simulink library "halin"  (R2021b)
settings: Solver=VariableStepAuto  StartTime=0.0  StopTime=10.0  RelTol=1e-3
undefined symbols (not defined in the file): TRUE
libraries: FVT_lib x177, hcu_lib x55
(part 17 of 17)

== system halin/HAL_IN/CAN4/zGW_SEAT1/PSEATSWVer ==
  PSEAT_SW_Ver : Inport
  UnitConverter : DataTypeConversion  OutDataTypeStr=uint16
  VHAL_PSEATSWVer_enum : Outport
  wires:
  UnitConverter/1 -> VHAL_PSEATSWVer_enum/1
  PSEAT_SW_Ver/1 -> UnitConverter/1

== system halin/HAL_IN/CAN4/zGW_SEAT1/PSEATVentSta ==
  PSEAT_Vent_Sta : Inport
  UnitConverter : DataTypeConversion  OutDataTypeStr=uint8
  VHAL_PSEATVentSta_enum : Outport
  wires:
  UnitConverter/1 -> VHAL_PSEATVentSta_enum/1
  PSEAT_Vent_Sta/1 -> UnitConverter/1

== system halin/HAL_IN/CAN4/zGW_SEAT1/PSEATheatersta ==
  PSEAT_heater_sta : Inport
  UnitConverter : DataTypeConversion  OutDataTypeStr=uint8
  VHAL_PSEATheatersta_enum : Outport
  wires:
  UnitConverter/1 -> VHAL_PSEATheatersta_enum/1
  PSEAT_heater_sta/1 -> UnitConverter/1

== system halin/HAL_IN/CAN5/TBOX1/CbnPreACEnaReq ==
  CbnPreACEnaReq : Inport
  UnitConverter : DataTypeConversion  OutDataTypeStr=uint8
  VHAL_CbnPreACEnaReq_enum : Outport
  wires:
  UnitConverter/1 -> VHAL_CbnPreACEnaReq_enum/1
  CbnPreACEnaReq/1 -> UnitConverter/1

== system halin/HAL_IN/CAN5/TBOX1/PowerOffTSet ==
  PowerOff_T_Set : Inport
  UnitConverter : DataTypeConversion  OutDataTypeStr=uint8
  convert_in : FVT_lib/hal/convert_in  gain=1  offset=1
  VHAL_PowerOffTSet_cnt : Outport
  wires:
  convert_in/1 -> VHAL_PowerOffTSet_cnt/1
  UnitConverter/1 -> convert_in/1
  PowerOff_T_Set/1 -> UnitConverter/1

== system halin/HAL_IN/CAN5/TBOX1/ReDoorLock ==
  Re_DoorLock : Inport
  UnitConverter : DataTypeConversion  OutDataTypeStr=uint16
  VHAL_ReDoorLock_enum : Outport
  wires:
  UnitConverter/1 -> VHAL_ReDoorLock_enum/1
  Re_DoorLock/1 -> UnitConverter/1

== system halin/HAL_IN/CAN5/TBOX1/ReOutsideMirror ==
  ReOutsideMirror : Inport
  UnitConverter : DataTypeConversion  OutDataTypeStr=uint8
  VHAL_ReOutsideMirror_enum : Outport
  wires:
  UnitConverter/1 -> VHAL_ReOutsideMirror_enum/1
  ReOutsideMirror/1 -> UnitConverter/1

== system halin/HAL_IN/CAN5/TBOX1/RePwrReqTbox ==
  Re_PwrReqTbox : Inport
  UnitConverter : DataTypeConversion  OutDataTypeStr=uint8
  VHAL_RePwrReqTbox_enum : Outport
  wires:
  UnitConverter/1 -> VHAL_RePwrReqTbox_enum/1
  Re_PwrReqTbox/1 -> UnitConverter/1

== system halin/HAL_IN/CAN5/TBOX1/ReRadio ==
  Re_Radio : Inport
  UnitConverter : DataTypeConversion  OutDataTypeStr=uint8
  VHAL_ReRadio_flg : Outport
  wires:
  UnitConverter/1 -> VHAL_ReRadio_flg/1
  Re_Radio/1 -> UnitConverter/1

== system halin/HAL_IN/CAN5/TBOX1/RemoteACTemp ==
  Remote_ACTemp : Inport
  UnitConverter : DataTypeConversion  OutDataTypeStr=uint8
  convert_in : FVT_lib/hal/convert_in  gain=0.5  offset=17
  VHAL_RemoteACTemp_C : Outport
  wires:
  convert_in/1 -> VHAL_RemoteACTemp_C/1
  UnitConverter/1 -> convert_in/1
  Remote_ACTemp/1 -> UnitConverter/1

== system halin/HAL_IN/CAN5/TBOX1/RemoteAutoReq ==
  Remote_AutoReq : Inport
  UnitConverter : DataTypeConversion  OutDataTypeStr=uint8
  VHAL_RemoteAutoReq_flg : Outport
  wires:
  UnitConverter/1 -> VHAL_RemoteAutoReq_flg/1
  Remote_AutoReq/1 -> UnitConverter/1

== system halin/HAL_IN/CAN5/TBOX1/TBOXNETSIGSTR ==
  TBOX_NET_SIG_STR : Inport
  UnitConverter : DataTypeConversion  OutDataTypeStr=uint8
  VHAL_TBOXNETSIGSTR_enum : Outport
  wires:
  UnitConverter/1 -> VHAL_TBOXNETSIGSTR_enum/1
  TBOX_NET_SIG_STR/1 -> UnitConverter/1

== system halin/HAL_IN/CAN5/TBOX1/TBOXRemotePW ==
  TBOX_Remote_PW : Inport
  UnitConverter : DataTypeConversion  OutDataTypeStr=uint8
  VHAL_TBOXRemotePW_enum : Outport
  wires:
  UnitConverter/1 -> VHAL_TBOXRemotePW_enum/1
  TBOX_Remote_PW/1 -> UnitConverter/1

== system halin/HAL_IN/CAN5/TBOX1/TBOXTESTSTATUS ==
  TBOX_TEST_STATUS : Inport
  UnitConverter : DataTypeConversion  OutDataTypeStr=uint8
  VHAL_TBOXTESTSTATUS_enum : Outport
  wires:
  UnitConverter/1 -> VHAL_TBOXTESTSTATUS_enum/1
  TBOX_TEST_STATUS/1 -> UnitConverter/1

== system halin/HAL_IN/CAN5/TBOX2/TimeSyncFromBSDay ==
  TimeSyncFromBS_Day : Inport
  UnitConverter : DataTypeConversion  OutDataTypeStr=uint8
  VHAL_TimeSyncFromBSDay_DAY : Outport
  wires:
  UnitConverter/1 -> VHAL_TimeSyncFromBSDay_DAY/1
  TimeSyncFromBS_Day/1 -> UnitConverter/1

== system halin/HAL_IN/CAN5/TBOX2/TimeSyncFromBSHour ==
  TimeSyncFromBS_Hour : Inport
  UnitConverter : DataTypeConversion  OutDataTypeStr=uint8
  VHAL_TimeSyncFromBSHour_hr : Outport
  wires:
  UnitConverter/1 -> VHAL_TimeSyncFromBSHour_hr/1
  TimeSyncFromBS_Hour/1 -> UnitConverter/1

== system halin/HAL_IN/CAN5/TBOX2/TimeSyncFromBSMinute ==
  TimeSyncFromBS_Minute : Inport
  UnitConverter : DataTypeConversion  OutDataTypeStr=uint8
  VHAL_TimeSyncFromBSMinute_min : Outport
  wires:
  UnitConverter/1 -> VHAL_TimeSyncFromBSMinute_min/1
  TimeSyncFromBS_Minute/1 -> UnitConverter/1

== system halin/HAL_IN/CAN5/TBOX2/TimeSyncFromBSMonth ==
  TimeSyncFromBS_Month : Inport
  UnitConverter : DataTypeConversion  OutDataTypeStr=uint8
  VHAL_TimeSyncFromBSMonth_MONTH : Outport
  wires:
  UnitConverter/1 -> VHAL_TimeSyncFromBSMonth_MONTH/1
  TimeSyncFromBS_Month/1 -> UnitConverter/1

== system halin/HAL_IN/CAN5/TBOX2/TimeSyncFromBSSecond ==
  TimeSyncFromBS_Second : Inport
  UnitConverter : DataTypeConversion  OutDataTypeStr=uint8
  VHAL_TimeSyncFromBSSecond_s : Outport
  wires:
  UnitConverter/1 -> VHAL_TimeSyncFromBSSecond_s/1
  TimeSyncFromBS_Second/1 -> UnitConverter/1

== system halin/HAL_IN/CAN5/TBOX2/TimeSyncFromBSYear ==
  TimeSyncFromBS_Year : Inport
  UnitConverter : DataTypeConversion  OutDataTypeStr=uint8
  convert_in : FVT_lib/hal/convert_in  gain=1  offset=2000
  VHAL_TimeSyncFromBSYear_YEAR : Outport
  wires:
  convert_in/1 -> VHAL_TimeSyncFromBSYear_YEAR/1
  UnitConverter/1 -> convert_in/1
  TimeSyncFromBS_Year/1 -> UnitConverter/1

== system halin/HAL_IN/CAN5/TBOX3/ChargePercentSet ==
  Charge_Percent_Set : Inport
  UnitConverter : DataTypeConversion  OutDataTypeStr=uint8
  VHAL_ChargePercentSet_pct : Outport
  wires:
  UnitConverter/1 -> VHAL_ChargePercentSet_pct/1
  Charge_Percent_Set/1 -> UnitConverter/1

== system halin/HAL_IN/CAN5/TBOX3/ReserveChargeOFFDay ==
  ReserveChargeOFF_Day : Inport
  UnitConverter : DataTypeConversion  OutDataTypeStr=uint8
  VHAL_ReserveChargeOFFDay_DAY : Outport
  wires:
  UnitConverter/1 -> VHAL_ReserveChargeOFFDay_DAY/1
  ReserveChargeOFF_Day/1 -> UnitConverter/1

== system halin/HAL_IN/CAN5/TBOX3/ReserveChargeOFFHour ==
  ReserveChargeOFF_Hour : Inport
  UnitConverter : DataTypeConversion  OutDataTypeStr=uint8
  VHAL_ReserveChargeOFFHour_hr : Outport
  wires:
  UnitConverter/1 -> VHAL_ReserveChargeOFFHour_hr/1
  ReserveChargeOFF_Hour/1 -> UnitConverter/1

== system halin/HAL_IN/CAN5/TBOX3/ReserveChargeOFFMinute ==
  ReserveChargeOFF_Minute : Inport
  UnitConverter : DataTypeConversion  OutDataTypeStr=uint8
  VHAL_ReserveChargeOFFMinute_min : Outport
  wires:
  UnitConverter/1 -> VHAL_ReserveChargeOFFMinute_min/1
  ReserveChargeOFF_Minute/1 -> UnitConverter/1

== system halin/HAL_IN/CAN5/TBOX3/ReserveChargeOFFMonth ==
  ReserveChargeOFF_Month : Inport
  UnitConverter : DataTypeConversion  OutDataTypeStr=uint8
  VHAL_ReserveChargeOFFMonth_MONTH : Outport
  wires:
  UnitConverter/1 -> VHAL_ReserveChargeOFFMonth_MONTH/1
  ReserveChargeOFF_Month/1 -> UnitConverter/1

== system halin/HAL_IN/CAN5/TBOX3/ReserveChargeOFFYear ==
  ReserveChargeOFF_Year : Inport
  UnitConverter : DataTypeConversion  OutDataTypeStr=uint8
  convert_in : FVT_lib/hal/convert_in  gain=1  offset=2000
  VHAL_ReserveChargeOFFYear_YEAR : Outport
  wires:
  convert_in/1 -> VHAL_ReserveChargeOFFYear_YEAR/1
  UnitConverter/1 -> convert_in/1
  ReserveChargeOFF_Year/1 -> UnitConverter/1

== system halin/HAL_IN/CAN5/TBOX3/ReserveChargeOnDay ==
  ReserveChargeOn_Day : Inport
  UnitConverter : DataTypeConversion  OutDataTypeStr=uint8
  VHAL_ReserveChargeOnDay_DAY : Outport
  wires:
  UnitConverter/1 -> VHAL_ReserveChargeOnDay_DAY/1
  ReserveChargeOn_Day/1 -> UnitConverter/1

== system halin/HAL_IN/CAN5/TBOX3/ReserveChargeOnHour ==
  ReserveChargeOn_Hour : Inport
  UnitConverter : DataTypeConversion  OutDataTypeStr=uint8
  VHAL_ReserveChargeOnHour_hr : Outport
  wires:
  UnitConverter/1 -> VHAL_ReserveChargeOnHour_hr/1
  ReserveChargeOn_Hour/1 -> UnitConverter/1

== system halin/HAL_IN/CAN5/TBOX3/ReserveChargeOnMinute ==
  ReserveChargeOn_Minute : Inport
  UnitConverter : DataTypeConversion  OutDataTypeStr=uint8
  VHAL_ReserveChargeOnMinute_min : Outport
  wires:
  UnitConverter/1 -> VHAL_ReserveChargeOnMinute_min/1
  ReserveChargeOn_Minute/1 -> UnitConverter/1

== system halin/HAL_IN/CAN5/TBOX3/ReserveChargeOnMonth ==
  ReserveChargeOn_Month : Inport
  UnitConverter : DataTypeConversion  OutDataTypeStr=uint8
  VHAL_ReserveChargeOnMonth_MONTH : Outport
  wires:
  UnitConverter/1 -> VHAL_ReserveChargeOnMonth_MONTH/1
  ReserveChargeOn_Month/1 -> UnitConverter/1

== system halin/HAL_IN/CAN5/TBOX3/ReserveChargeOnYear ==
  ReserveChargeOn_Year : Inport
  UnitConverter : DataTypeConversion  OutDataTypeStr=uint8
  convert_in : FVT_lib/hal/convert_in  gain=1  offset=2000
  VHAL_ReserveChargeOnYear_YEAR : Outport
  wires:
  convert_in/1 -> VHAL_ReserveChargeOnYear_YEAR/1
  UnitConverter/1 -> convert_in/1
  ReserveChargeOn_Year/1 -> UnitConverter/1

== system halin/HAL_IN/CAN5/TBOX3/TBOXHWVER ==
  TBOX_HW_VER : Inport
  UnitConverter : DataTypeConversion  OutDataTypeStr=uint32
  VHAL_TBOXHWVER_enum : Outport
  wires:
  UnitConverter/1 -> VHAL_TBOXHWVER_enum/1
  TBOX_HW_VER/1 -> UnitConverter/1

== system halin/HAL_IN/CAN5/TBOX3/TBOXSWVER ==
  TBOX_SW_VER : Inport
  UnitConverter : DataTypeConversion  OutDataTypeStr=uint32
  VHAL_TBOXSWVER_enum : Outport
  wires:
  UnitConverter/1 -> VHAL_TBOXSWVER_enum/1
  TBOX_SW_VER/1 -> UnitConverter/1

== system halin/HAL_IN/CAN6/FCM1/ACCComfortBandLower ==
  ACC_ComfortBandLower : Inport
  UnitConverter : DataTypeConversion  OutDataTypeStr=uint16
  convert_in : FVT_lib/hal/convert_in  gain=0.05  offset=-15
  VHAL_ACCComfortBandLower_mps2 : Outport
  wires:
  convert_in/1 -> VHAL_ACCComfortBandLower_mps2/1
  UnitConverter/1 -> convert_in/1
  ACC_ComfortBandLower/1 -> UnitConverter/1

== system halin/HAL_IN/CAN6/FCM1/ACCComfortBandUpper ==
  ACC_ComfortBandUpper : Inport
  UnitConverter : DataTypeConversion  OutDataTypeStr=uint16
  convert_in : FVT_lib/hal/convert_in  gain=0.05  offset=-15
  VHAL_ACCComfortBandUpper_mps2 : Outport
  wires:
  convert_in/1 -> VHAL_ACCComfortBandUpper_mps2/1
  UnitConverter/1 -> convert_in/1
  ACC_ComfortBandUpper/1 -> UnitConverter/1

== system halin/HAL_IN/CAN6/FCM1/ACCJerkLowerLimit ==
  ACC_JerkLowerLimit : Inport
  UnitConverter : DataTypeConversion  OutDataTypeStr=uint8
  convert_in : FVT_lib/hal/convert_in  gain=0.1  offset=-6
  VHAL_ACCJerkLowerLimit_mps3 : Outport
  wires:
  convert_in/1 -> VHAL_ACCJerkLowerLimit_mps3/1
  UnitConverter/1 -> convert_in/1
  ACC_JerkLowerLimit/1 -> UnitConverter/1

== system halin/HAL_IN/CAN6/FCM1/ACCJerkUpperLimit ==
  ACC_JerkUpperLimit : Inport
  UnitConverter : DataTypeConversion  OutDataTypeStr=uint8
  convert_in : FVT_lib/hal/convert_in  gain=0.1  offset=-6
  VHAL_ACCJerkUpperLimit_mps3 : Outport
  wires:
  convert_in/1 -> VHAL_ACCJerkUpperLimit_mps3/1
  UnitConverter/1 -> convert_in/1
  ACC_JerkUpperLimit/1 -> UnitConverter/1

== system halin/HAL_IN/CAN6/FCM1/ACCObjDist ==
  ACC_ObjDist : Inport
  UnitConverter : DataTypeConversion  OutDataTypeStr=uint16
  convert_in : FVT_lib/hal/convert_in  gain=0.1  offset=0
  VHAL_ACCObjDist_m : Outport
  wires:
  convert_in/1 -> VHAL_ACCObjDist_m/1
  UnitConverter/1 -> convert_in/1
  ACC_ObjDist/1 -> UnitConverter/1

== system halin/HAL_IN/CAN6/FCM1/ACCObjDstLvl ==
  ACC_ObjDstLvl : Inport
  UnitConverter : DataTypeConversion  OutDataTypeStr=uint8
  VHAL_ACCObjDstLvl_enum : Outport
  wires:
  UnitConverter/1 -> VHAL_ACCObjDstLvl_enum/1
  ACC_ObjDstLvl/1 -> UnitConverter/1

== system halin/HAL_IN/CAN6/FCM1/ACCObjRelSpd ==
  ACC_ObjRelSpd : Inport
  UnitConverter : DataTypeConversion  OutDataTypeStr=uint16
  convert_in : FVT_lib/hal/convert_in  gain=0.1  offset=-100
  VHAL_ACCObjRelSpd_mps : Outport
  wires:
  convert_in/1 -> VHAL_ACCObjRelSpd_mps/1
  UnitConverter/1 -> convert_in/1
  ACC_ObjRelSpd/1 -> UnitConverter/1

== system halin/HAL_IN/CAN6/FCM1/ACCRequiredAccel ==
  ACC_RequiredAccel : Inport
  UnitConverter : DataTypeConversion  OutDataTypeStr=uint16
  convert_in : FVT_lib/hal/convert_in  gain=0.05  offset=-15
  VHAL_ACCRequiredAccel_mps2 : Outport
  wires:
  convert_in/1 -> VHAL_ACCRequiredAccel_mps2/1
  UnitConverter/1 -> convert_in/1
  ACC_RequiredAccel/1 -> UnitConverter/1

== system halin/HAL_IN/CAN6/FCM1/ACCTakeoverReq ==
  ACC_TakeoverReq : Inport
  UnitConverter : DataTypeConversion  OutDataTypeStr=uint8
  VHAL_ACCTakeoverReq_flg : Outport
  wires:
  UnitConverter/1 -> VHAL_ACCTakeoverReq_flg/1
  ACC_TakeoverReq/1 -> UnitConverter/1

== system halin/HAL_IN/CAN6/FCM1/ACCVehHoldReq ==
  ACC_VehHoldReq : Inport
  UnitConverter : DataTypeConversion  OutDataTypeStr=uint8
  VHAL_ACCVehHoldReq_flg : Outport
  wires:
  UnitConverter/1 -> VHAL_ACCVehHoldReq_flg/1
  ACC_VehHoldReq/1 -> UnitConverter/1

== system halin/HAL_IN/CAN6/FCM1/ADASACCSta ==
  ADAS_ACC_Sta : Inport
  UnitConverter : DataTypeConversion  OutDataTypeStr=uint8
  VHAL_ADASACCSta_enum : Outport
  wires:
  UnitConverter/1 -> VHAL_ADASACCSta_enum/1
  ADAS_ACC_Sta/1 -> UnitConverter/1

== system halin/HAL_IN/CAN6/FCM1/ADASAEBReq ==
  ADAS_AEBReq : Inport
  UnitConverter : DataTypeConversion  OutDataTypeStr=uint8
  VHAL_ADASAEBReq_enum : Outport
  wires:
  UnitConverter/1 -> VHAL_ADASAEBReq_enum/1
  ADAS_AEBReq/1 -> UnitConverter/1

== system halin/HAL_IN/CAN6/FCM1/ADASAEBSta ==
  ADAS_AEB_Sta : Inport
  UnitConverter : DataTypeConversion  OutDataTypeStr=uint8
  VHAL_ADASAEBSta_enum : Outport
  wires:
  UnitConverter/1 -> VHAL_ADASAEBSta_enum/1
  ADAS_AEB_Sta/1 -> UnitConverter/1

== system halin/HAL_IN/CAN6/FCM1/ADASCAMSpdLim ==
  ADAS_CAM_SpdLim : Inport
  UnitConverter : DataTypeConversion  OutDataTypeStr=uint8
  VHAL_ADASCAMSpdLim_enum : Outport
  wires:
  UnitConverter/1 -> VHAL_ADASCAMSpdLim_enum/1
  ADAS_CAM_SpdLim/1 -> UnitConverter/1

== system halin/HAL_IN/CAN6/FCM1/ADASDBSReq ==
  ADAS_DBSReq : Inport
  UnitConverter : DataTypeConversion  OutDataTypeStr=uint8
  VHAL_ADASDBSReq_enum : Outport
  wires:
  UnitConverter/1 -> VHAL_ADASDBSReq_enum/1
  ADAS_DBSReq/1 -> UnitConverter/1

== system halin/HAL_IN/CAN6/FCM1/ADASFCWMute ==
  ADAS_FCW_Mute : Inport
  UnitConverter : DataTypeConversion  OutDataTypeStr=uint8
  VHAL_ADASFCWMute_flg : Outport
  wires:
  UnitConverter/1 -> VHAL_ADASFCWMute_flg/1
  ADAS_FCW_Mute/1 -> UnitConverter/1

== system halin/HAL_IN/CAN6/FCM1/ADASFCWSta ==
  ADAS_FCW_Sta : Inport
  UnitConverter : DataTypeConversion  OutDataTypeStr=uint8
  VHAL_ADASFCWSta_enum : Outport
  wires:
  UnitConverter/1 -> VHAL_ADASFCWSta_enum/1
  ADAS_FCW_Sta/1 -> UnitConverter/1

== system halin/HAL_IN/CAN6/FCM1/ADASFaultSta ==
  ADAS_FaultSta : Inport
  UnitConverter : DataTypeConversion  OutDataTypeStr=uint8
  VHAL_ADASFaultSta_flg : Outport
  wires:
  UnitConverter/1 -> VHAL_ADASFaultSta_flg/1
  ADAS_FaultSta/1 -> UnitConverter/1

== system halin/HAL_IN/CAN6/FCM1/ADASFltWrnReq ==
  ADAS_FltWrnReq : Inport
  UnitConverter : DataTypeConversion  OutDataTypeStr=uint8
  VHAL_ADASFltWrnReq_flg : Outport
  wires:
  UnitConverter/1 -> VHAL_ADASFltWrnReq_flg/1
  ADAS_FltWrnReq/1 -> UnitConverter/1

== system halin/HAL_IN/CAN6/FCM1/ADASForceIdle ==
  ADAS_ForceIdle : Inport
  UnitConverter : DataTypeConversion  OutDataTypeStr=uint8
  VHAL_ADASForceIdle_flg : Outport
  wires:
  UnitConverter/1 -> VHAL_ADASForceIdle_flg/1
  ADAS_ForceIdle/1 -> UnitConverter/1

== system halin/HAL_IN/CAN6/FCM1/ADASISASta ==
  ADAS_ISA_Sta : Inport
  UnitConverter : DataTypeConversion  OutDataTypeStr=uint8
  VHAL_ADASISASta_enum : Outport
  wires:
  UnitConverter/1 -> VHAL_ADASISASta_enum/1
  ADAS_ISA_Sta/1 -> UnitConverter/1

== system halin/HAL_IN/CAN6/FCM1/ADASLDWMute ==
  ADAS_LDW_Mute : Inport
  UnitConverter : DataTypeConversion  OutDataTypeStr=uint8
  VHAL_ADASLDWMute_flg : Outport
  wires:
  UnitConverter/1 -> VHAL_ADASLDWMute_flg/1
  ADAS_LDW_Mute/1 -> UnitConverter/1

== system halin/HAL_IN/CAN6/FCM1/ADASLDWSta ==
  ADAS_LDW_Sta : Inport
  UnitConverter : DataTypeConversion  OutDataTypeStr=uint8
  VHAL_ADASLDWSta_enum : Outport
  wires:
  UnitConverter/1 -> VHAL_ADASLDWSta_enum/1
  ADAS_LDW_Sta/1 -> UnitConverter/1

== system halin/HAL_IN/CAN6/FCM1/ADASLFCHandsOffWarning ==
  ADAS_LFC_Hands_Off_Warning : Inport
  UnitConverter : DataTypeConversion  OutDataTypeStr=uint8
  VHAL_ADASLFCHandsOffWarning_enum : Outport
  wires:
  UnitConverter/1 -> VHAL_ADASLFCHandsOffWarning_enum/1
  ADAS_LFC_Hands_Off_Warning/1 -> UnitConverter/1

== system halin/HAL_IN/CAN6/FCM1/ADASLFCSta ==
  ADAS_LFC_Sta : Inport
  UnitConverter : DataTypeConversion  OutDataTypeStr=uint8
  VHAL_ADASLFCSta_enum : Outport
  wires:
  UnitConverter/1 -> VHAL_ADASLFCSta_enum/1
  ADAS_LFC_Sta/1 -> UnitConverter/1

== system halin/HAL_IN/CAN6/FCM1/ADASLFCWarnSound ==
  ADAS_LFC_Warn_Sound : Inport
  UnitConverter : DataTypeConversion  OutDataTypeStr=uint16
  VHAL_ADASLFCWarnSound_enum : Outport
  wires:
  UnitConverter/1 -> VHAL_ADASLFCWarnSound_enum/1
  ADAS_LFC_Warn_Sound/1 -> UnitConverter/1

== system halin/HAL_IN/CAN6/FCM1/ADASLKASta ==
  ADAS_LKA_Sta : Inport
  UnitConverter : DataTypeConversion  OutDataTypeStr=uint16
  VHAL_ADASLKASta_enum : Outport
  wires:
  UnitConverter/1 -> VHAL_ADASLKASta_enum/1
  ADAS_LKA_Sta/1 -> UnitConverter/1

== system halin/HAL_IN/CAN6/FCM1/ADASLaneModeL ==
  ADAS_LaneModeL : Inport
  UnitConverter : DataTypeConversion  OutDataTypeStr=uint16
  VHAL_ADASLaneModeL_enum : Outport
  wires:
  UnitConverter/1 -> VHAL_ADASLaneModeL_enum/1
  ADAS_LaneModeL/1 -> UnitConverter/1

== system halin/HAL_IN/CAN6/FCM1/ADASLaneModeR ==
  ADAS_LaneModeR : Inport
  UnitConverter : DataTypeConversion  OutDataTypeStr=uint8
  VHAL_ADASLaneModeR_enum : Outport
  wires:
  UnitConverter/1 -> VHAL_ADASLaneModeR_enum/1
  ADAS_LaneModeR/1 -> UnitConverter/1

== system halin/HAL_IN/CAN6/FCM1/ADASLanecurveL ==
  ADAS_Lane_curveL : Inport
  UnitConverter : DataTypeConversion  OutDataTypeStr=uint8
  convert_in : FVT_lib/hal/convert_in  gain=0.0005  offset=-0.03
  VHAL_ADASLanecurveL_raw32 : Outport
  wires:
  convert_in/1 -> VHAL_ADASLanecurveL_raw32/1
  UnitConverter/1 -> convert_in/1
  ADAS_Lane_curveL/1 -> UnitConverter/1

== system halin/HAL_IN/CAN6/FCM1/ADASLanecurveR ==
  ADAS_Lane_curveR : Inport
  UnitConverter : DataTypeConversion  OutDataTypeStr=uint8
  convert_in : FVT_lib/hal/convert_in  gain=0.0005  offset=-0.03
  VHAL_ADASLanecurveR_raw32 : Outport
  wires:
  convert_in/1 -> VHAL_ADASLanecurveR_raw32/1
  UnitConverter/1 -> convert_in/1
  ADAS_Lane_curveR/1 -> UnitConverter/1

== system halin/HAL_IN/CAN6/FCM1/ADASLanetypeL ==
  ADAS_LanetypeL : Inport
  UnitConverter : DataTypeConversion  OutDataTypeStr=uint16
  VHAL_ADASLanetypeL_enum : Outport
  wires:
  UnitConverter/1 -> VHAL_ADASLanetypeL_enum/1
  ADAS_LanetypeL/1 -> UnitConverter/1

== system halin/HAL_IN/CAN6/FCM1/ADASLanetypeR ==
  ADAS_LanetypeR : Inport
  UnitConverter : DataTypeConversion  OutDataTypeStr=uint8
  VHAL_ADASLanetypeR_enum : Outport
  wires:
  UnitConverter/1 -> VHAL_ADASLanetypeR_enum/1
  ADAS_LanetypeR/1 -> UnitConverter/1

== system halin/HAL_IN/CAN6/FCM1/ADASSLIFSpdLim ==
  ADAS_SLIF_SpdLim : Inport
  UnitConverter : DataTypeConversion  OutDataTypeStr=uint8
  VHAL_ADASSLIFSpdLim_enum : Outport
  wires:
  UnitConverter/1 -> VHAL_ADASSLIFSpdLim_enum/1
  ADAS_SLIF_SpdLim/1 -> UnitConverter/1

== system halin/HAL_IN/CAN6/FCM1/ADASSLIFSta ==
  ADAS_SLIF_Sta : Inport
  UnitConverter : DataTypeConversion  OutDataTypeStr=uint8
  VHAL_ADASSLIFSta_enum : Outport
  wires:
  UnitConverter/1 -> VHAL_ADASSLIFSta_enum/1
  ADAS_SLIF_Sta/1 -> UnitConverter/1

== system halin/HAL_IN/CAN6/FCM1/ADASShftPosnReq ==
  ADAS_ShftPosnReq : Inport
  UnitConverter : DataTypeConversion  OutDataTypeStr=uint8
  VHAL_ADASShftPosnReq_enum : Outport
  wires:
  UnitConverter/1 -> VHAL_ADASShftPosnReq_enum/1
  ADAS_ShftPosnReq/1 -> UnitConverter/1

== system halin/HAL_IN/CAN6/FCM1/ADASShftPosnReqA ==
  ADAS_ShftPosnReq_A : Inport
  UnitConverter : DataTypeConversion  OutDataTypeStr=uint8
  VHAL_ADASShftPosnReqA_flg : Outport
  wires:
  UnitConverter/1 -> VHAL_ADASShftPosnReqA_flg/1
  ADAS_ShftPosnReq_A/1 -> UnitConverter/1

== system halin/HAL_IN/CAN6/FCM1/ADASVehSpdLim ==
  ADAS_VehSpdLim : Inport
  UnitConverter : DataTypeConversion  OutDataTypeStr=uint8
  VHAL_ADASVehSpdLim_enum : Outport
  wires:
  UnitConverter/1 -> VHAL_ADASVehSpdLim_enum/1
  ADAS_VehSpdLim/1 -> UnitConverter/1

== system halin/HAL_IN/CAN6/FCM1/ADASWarningMsg ==
  ADAS_WarningMsg : Inport
  UnitConverter : DataTypeConversion  OutDataTypeStr=uint8
  VHAL_ADASWarningMsg_enum : Outport
  wires:
  UnitConverter/1 -> VHAL_ADASWarningMsg_enum/1
  ADAS_WarningMsg/1 -> UnitConverter/1

== system halin/HAL_IN/CAN6/FCM1/AEBVehHoldReq ==
  AEB_VehHoldReq : Inport
  UnitConverter : DataTypeConversion  OutDataTypeStr=uint8
  VHAL_AEBVehHoldReq_flg : Outport
  wires:
  UnitConverter/1 -> VHAL_AEBVehHoldReq_flg/1
  AEB_VehHoldReq/1 -> UnitConverter/1

== system halin/HAL_IN/CAN6/FCM1/CameraBlockage ==
  CameraBlockage : Inport
  UnitConverter : DataTypeConversion  OutDataTypeStr=uint8
  VHAL_CameraBlockage_flg : Outport
  wires:
  UnitConverter/1 -> VHAL_CameraBlockage_flg/1
  CameraBlockage/1 -> UnitConverter/1

== system halin/HAL_IN/CAN6/FCM1/FCM1Checksum ==
  FCM1_Checksum : Inport
  UnitConverter : DataTypeConversion  OutDataTypeStr=uint8
  VHAL_FCM1Checksum_enum : Outport
  wires:
  UnitConverter/1 -> VHAL_FCM1Checksum_enum/1
  FCM1_Checksum/1 -> UnitConverter/1

== system halin/HAL_IN/CAN6/FCM1/FCM1LifeCount ==
  FCM1_LifeCount : Inport
  UnitConverter : DataTypeConversion  OutDataTypeStr=uint8
  VHAL_FCM1LifeCount_enum : Outport
  wires:
  UnitConverter/1 -> VHAL_FCM1LifeCount_enum/1
  FCM1_LifeCount/1 -> UnitConverter/1

== system halin/HAL_IN/CAN6/FCM1/FCMACCmode ==
  FCM_ACCmode : Inport
  UnitConverter : DataTypeConversion  OutDataTypeStr=uint8
  VHAL_FCMACCmode_enum : Outport
  wires:
  UnitConverter/1 -> VHAL_FCMACCmode_enum/1
  FCM_ACCmode/1 -> UnitConverter/1

== system halin/HAL_IN/CAN6/FCM1/FCMLKAStrToqReq ==
  FCM_LKA_StrToqReq : Inport
  UnitConverter : DataTypeConversion  OutDataTypeStr=uint16
  convert_in : FVT_lib/hal/convert_in  gain=0.008  offset=-8
  VHAL_FCMLKAStrToqReq_Nm : Outport
  wires:
  convert_in/1 -> VHAL_FCMLKAStrToqReq_Nm/1
  UnitConverter/1 -> convert_in/1
  FCM_LKA_StrToqReq/1 -> UnitConverter/1

== system halin/HAL_IN/CAN6/FCM1/FCMLKATOIAct ==
  FCM_LKA_TOIAct : Inport
  UnitConverter : DataTypeConversion  OutDataTypeStr=uint8
  VHAL_FCMLKATOIAct_enum : Outport
  wires:
  UnitConverter/1 -> VHAL_FCMLKATOIAct_enum/1
  FCM_LKA_TOIAct/1 -> UnitConverter/1

== system halin/HAL_IN/CAN6/FCM1/FCMLKATOIFault ==
  FCM_LKA_TOIFault : Inport
  UnitConverter : DataTypeConversion  OutDataTypeStr=uint8
  VHAL_FCMLKATOIFault_flg : Outport
  wires:
  UnitConverter/1 -> VHAL_FCMLKATOIFault_flg/1
  FCM_LKA_TOIFault/1 -> UnitConverter/1

== system halin/HAL_IN/CAN6/FCM1/ForceLowBeam ==
  ForceLowBeam : Inport
  UnitConverter : DataTypeConversion  OutDataTypeStr=uint8
  VHAL_ForceLowBeam_enum : Outport
  wires:
  UnitConverter/1 -> VHAL_ForceLowBeam_enum/1
  ForceLowBeam/1 -> UnitConverter/1

== system halin/HAL_IN/CAN6/FCM1/HazardWarningReq ==
  HazardWarningReq : Inport
  UnitConverter : DataTypeConversion  OutDataTypeStr=uint8
  VHAL_HazardWarningReq_flg : Outport
  wires:
  UnitConverter/1 -> VHAL_HazardWarningReq_flg/1
  HazardWarningReq/1 -> UnitConverter/1

== system halin/HAL_IN/CAN6/FCM1/ISAWarningMsg ==
  ISA_WarningMsg : Inport
  UnitConverter : DataTypeConversion  OutDataTypeStr=uint8
  VHAL_ISAWarningMsg_enum : Outport
  wires:
  UnitConverter/1 -> VHAL_ISAWarningMsg_enum/1
  ISA_WarningMsg/1 -> UnitConverter/1

== system halin/HAL_IN/CAN6/FCM1/LKAHODDisplayWarning ==
  LKA_HOD_Display_Warning : Inport
  UnitConverter : DataTypeConversion  OutDataTypeStr=uint8
  VHAL_LKAHODDisplayWarning_flg : Outport
  wires:
  UnitConverter/1 -> VHAL_LKAHODDisplayWarning_flg/1
  LKA_HOD_Display_Warning/1 -> UnitConverter/1

== system halin/HAL_IN/CAN6/FCM1/LKAHODSoundWarning ==
  LKA_HOD_Sound_Warning : Inport
  UnitConverter : DataTypeConversion  OutDataTypeStr=uint8
  VHAL_LKAHODSoundWarning_flg : Outport
  wires:
  UnitConverter/1 -> VHAL_LKAHODSoundWarning_flg/1
  LKA_HOD_Sound_Warning/1 -> UnitConverter/1

== system halin/HAL_IN/CAN6/FCM1/LVDAACCStatusInformation ==
  LVDA_ACCStatusInformation : Inport
  UnitConverter : DataTypeConversion  OutDataTypeStr=uint8
  VHAL_LVDAACCStatusInformation_flg : Outport
  wires:
  UnitConverter/1 -> VHAL_LVDAACCStatusInformation_flg/1
  LVDA_ACCStatusInformation/1 -> UnitConverter/1

== system halin/HAL_IN/CAN6/FCM1/LVDADisabled ==
  LVDA_Disabled : Inport
  UnitConverter : DataTypeConversion  OutDataTypeStr=uint8
  VHAL_LVDADisabled_flg : Outport
  wires:
  UnitConverter/1 -> VHAL_LVDADisabled_flg/1
  LVDA_Disabled/1 -> UnitConverter/1

== system halin/HAL_IN/CAN6/FCM1/LVDAFailinfo ==
  LVDA_Failinfo : Inport
  UnitConverter : DataTypeConversion  OutDataTypeStr=uint8
  VHAL_LVDAFailinfo_flg : Outport
  wires:
  UnitConverter/1 -> VHAL_LVDAFailinfo_flg/1
  LVDA_Failinfo/1 -> UnitConverter/1

== system halin/HAL_IN/CAN6/FCM1/LVDAMuteSta ==
  LVDA_Mute_Sta : Inport
  UnitConverter : DataTypeConversion  OutDataTypeStr=uint8
  VHAL_LVDAMuteSta_enum : Outport
  wires:
  UnitConverter/1 -> VHAL_LVDAMuteSta_enum/1
  LVDA_Mute_Sta/1 -> UnitConverter/1

== system halin/HAL_IN/CAN6/FCM1/LVDAWarning ==
  LVDA_Warning : Inport
  UnitConverter : DataTypeConversion  OutDataTypeStr=uint8
  VHAL_LVDAWarning_flg : Outport
  wires:
  UnitConverter/1 -> VHAL_LVDAWarning_flg/1
  LVDA_Warning/1 -> UnitConverter/1

== system halin/HAL_IN/CAN6/FCM1/LeftTurnLightReq ==
  LeftTurnLightReq : Inport
  UnitConverter : DataTypeConversion  OutDataTypeStr=uint8
  VHAL_LeftTurnLightReq_flg : Outport
  wires:
  UnitConverter/1 -> VHAL_LeftTurnLightReq_flg/1
  LeftTurnLightReq/1 -> UnitConverter/1

== system halin/HAL_IN/CAN6/FCM1/RightTurnLightReq ==
  RightTurnLightReq : Inport
  UnitConverter : DataTypeConversion  OutDataTypeStr=uint8
  VHAL_RightTurnLightReq_flg : Outport
  wires:
  UnitConverter/1 -> VHAL_RightTurnLightReq_flg/1
  RightTurnLightReq/1 -> UnitConverter/1

== system halin/HAL_IN/CAN6/FCM1/TargetType ==
  Target_Type : Inport
  UnitConverter : DataTypeConversion  OutDataTypeStr=uint16
  VHAL_TargetType_enum : Outport
  wires:
  UnitConverter/1 -> VHAL_TargetType_enum/1
  Target_Type/1 -> UnitConverter/1

== system halin/HAL_IN/CAN6/FCM1/TimeGapLevel ==
  TimeGapLevel : Inport
  UnitConverter : DataTypeConversion  OutDataTypeStr=uint8
  VHAL_TimeGapLevel_enum : Outport
  wires:
  UnitConverter/1 -> VHAL_TimeGapLevel_enum/1
  TimeGapLevel/1 -> UnitConverter/1

== system halin/HAL_IN/CAN6/FCM3/MELaneCurvDervLt ==
  ME_Lane_CurvDervLt : Inport
  UnitConverter : DataTypeConversion  OutDataTypeStr=uint16
  convert_in : FVT_lib/hal/convert_in  gain=4e-09  offset=-0.00013
  VHAL_MELaneCurvDervLt_raw32 : Outport
  wires:
  convert_in/1 -> VHAL_MELaneCurvDervLt_raw32/1
  UnitConverter/1 -> convert_in/1
  ME_Lane_CurvDervLt/1 -> UnitConverter/1

== system halin/HAL_IN/CAN6/FCM3/MELaneCurvDervLt2 ==
  ME_Lane_CurvDervLt2 : Inport
  UnitConverter : DataTypeConversion  OutDataTypeStr=uint16
  convert_in : FVT_lib/hal/convert_in  gain=4e-09  offset=-0.00013
  VHAL_MELaneCurvDervLt2_raw32 : Outport
  wires:
  convert_in/1 -> VHAL_MELaneCurvDervLt2_raw32/1
  UnitConverter/1 -> convert_in/1
  ME_Lane_CurvDervLt2/1 -> UnitConverter/1

== system halin/HAL_IN/CAN6/FCM3/MELaneCurvDervRt ==
  ME_Lane_CurvDervRt : Inport
  UnitConverter : DataTypeConversion  OutDataTypeStr=uint16
  convert_in : FVT_lib/hal/convert_in  gain=4e-09  offset=-0.00013
  VHAL_MELaneCurvDervRt_raw32 : Outport
  wires:
  convert_in/1 -> VHAL_MELaneCurvDervRt_raw32/1
  UnitConverter/1 -> convert_in/1
  ME_Lane_CurvDervRt/1 -> UnitConverter/1

== system halin/HAL_IN/CAN6/FCM3/MELaneCurvDervRt2 ==
  ME_Lane_CurvDervRt2 : Inport
  UnitConverter : DataTypeConversion  OutDataTypeStr=uint16
  convert_in : FVT_lib/hal/convert_in  gain=4e-09  offset=-0.00013
  VHAL_MELaneCurvDervRt2_raw32 : Outport
  wires:
  convert_in/1 -> VHAL_MELaneCurvDervRt2_raw32/1
  UnitConverter/1 -> convert_in/1
  ME_Lane_CurvDervRt2/1 -> UnitConverter/1

== system halin/HAL_IN/CAN6/FCM3/MELaneCurvLt ==
  ME_Lane_CurvLt : Inport
  UnitConverter : DataTypeConversion  OutDataTypeStr=uint16
  convert_in : FVT_lib/hal/convert_in  gain=1e-06  offset=-0.032
  VHAL_MELaneCurvLt_raw32 : Outport
  wires:
  convert_in/1 -> VHAL_MELaneCurvLt_raw32/1
  UnitConverter/1 -> convert_in/1
  ME_Lane_CurvLt/1 -> UnitConverter/1

== system halin/HAL_IN/CAN6/FCM3/MELaneCurvLt2 ==
  ME_Lane_CurvLt2 : Inport
  UnitConverter : DataTypeConversion  OutDataTypeStr=uint16
  convert_in : FVT_lib/hal/convert_in  gain=1e-06  offset=-0.032
  VHAL_MELaneCurvLt2_raw32 : Outport
  wires:
  convert_in/1 -> VHAL_MELaneCurvLt2_raw32/1
  UnitConverter/1 -> convert_in/1
  ME_Lane_CurvLt2/1 -> UnitConverter/1

== system halin/HAL_IN/CAN6/FCM3/MELaneCurvRt ==
  ME_Lane_CurvRt : Inport
  UnitConverter : DataTypeConversion  OutDataTypeStr=uint16
  convert_in : FVT_lib/hal/convert_in  gain=1e-06  offset=-0.032
  VHAL_MELaneCurvRt_raw32 : Outport
  wires:
  convert_in/1 -> VHAL_MELaneCurvRt_raw32/1
  UnitConverter/1 -> convert_in/1
  ME_Lane_CurvRt/1 -> UnitConverter/1

== system halin/HAL_IN/CAN6/FCM3/MELaneCurvRt2 ==
  ME_Lane_CurvRt2 : Inport
  UnitConverter : DataTypeConversion  OutDataTypeStr=uint16
  convert_in : FVT_lib/hal/convert_in  gain=1e-06  offset=-0.032
  VHAL_MELaneCurvRt2_raw32 : Outport
  wires:
  convert_in/1 -> VHAL_MELaneCurvRt2_raw32/1
  UnitConverter/1 -> convert_in/1
  ME_Lane_CurvRt2/1 -> UnitConverter/1

== system halin/HAL_IN/CAN6/FCM3/MELaneHeadAngLt ==
  ME_Lane_HeadAngLt : Inport
  UnitConverter : DataTypeConversion  OutDataTypeStr=uint16
  convert_in : FVT_lib/hal/convert_in  gain=0.001  offset=-0.5
  VHAL_MELaneHeadAngLt_radians : Outport
  wires:
  convert_in/1 -> VHAL_MELaneHeadAngLt_radians/1
  UnitConverter/1 -> convert_in/1
  ME_Lane_HeadAngLt/1 -> UnitConverter/1

== system halin/HAL_IN/CAN6/FCM3/MELaneHeadAngLt2 ==
  ME_Lane_HeadAngLt2 : Inport
  UnitConverter : DataTypeConversion  OutDataTypeStr=uint16
  convert_in : FVT_lib/hal/convert_in  gain=0.001  offset=-0.5
  VHAL_MELaneHeadAngLt2_radians : Outport
  wires:
  convert_in/1 -> VHAL_MELaneHeadAngLt2_radians/1
  UnitConverter/1 -> convert_in/1
  ME_Lane_HeadAngLt2/1 -> UnitConverter/1

== system halin/HAL_IN/CAN6/FCM3/MELaneHeadAngRt ==
  ME_Lane_HeadAngRt : Inport
  UnitConverter : DataTypeConversion  OutDataTypeStr=uint16
  convert_in : FVT_lib/hal/convert_in  gain=0.001  offset=-0.5
  VHAL_MELaneHeadAngRt_radians : Outport
  wires:
  convert_in/1 -> VHAL_MELaneHeadAngRt_radians/1
  UnitConverter/1 -> convert_in/1
  ME_Lane_HeadAngRt/1 -> UnitConverter/1

== system halin/HAL_IN/CAN6/FCM3/MELaneHeadAngRt2 ==
  ME_Lane_HeadAngRt2 : Inport
  UnitConverter : DataTypeConversion  OutDataTypeStr=uint16
  convert_in : FVT_lib/hal/convert_in  gain=0.001  offset=-0.5
  VHAL_MELaneHeadAngRt2_radians : Outport
  wires:
  convert_in/1 -> VHAL_MELaneHeadAngRt2_radians/1
  UnitConverter/1 -> convert_in/1
  ME_Lane_HeadAngRt2/1 -> UnitConverter/1

== system halin/HAL_IN/CAN6/FCM3/MELanePosLt ==
  ME_Lane_PosLt : Inport
  UnitConverter : DataTypeConversion  OutDataTypeStr=uint16
  convert_in : FVT_lib/hal/convert_in  gain=0.01  offset=-10
  VHAL_MELanePosLt_m : Outport
  wires:
  convert_in/1 -> VHAL_MELanePosLt_m/1
  UnitConverter/1 -> convert_in/1
  ME_Lane_PosLt/1 -> UnitConverter/1

== system halin/HAL_IN/CAN6/FCM3/MELanePosLt2 ==
  ME_Lane_PosLt2 : Inport
  UnitConverter : DataTypeConversion  OutDataTypeStr=uint16
  convert_in : FVT_lib/hal/convert_in  gain=0.01  offset=-10
  VHAL_MELanePosLt2_m : Outport
  wires:
  convert_in/1 -> VHAL_MELanePosLt2_m/1
  UnitConverter/1 -> convert_in/1
  ME_Lane_PosLt2/1 -> UnitConverter/1

== system halin/HAL_IN/CAN6/FCM3/MELanePosRt ==
  ME_Lane_PosRt : Inport
  UnitConverter : DataTypeConversion  OutDataTypeStr=uint16
  convert_in : FVT_lib/hal/convert_in  gain=0.01  offset=-10
  VHAL_MELanePosRt_m : Outport
  wires:
  convert_in/1 -> VHAL_MELanePosRt_m/1
  UnitConverter/1 -> convert_in/1
  ME_Lane_PosRt/1 -> UnitConverter/1

== system halin/HAL_IN/CAN6/FCM3/MELanePosRt2 ==
  ME_Lane_PosRt2 : Inport
  UnitConverter : DataTypeConversion  OutDataTypeStr=uint16
  convert_in : FVT_lib/hal/convert_in  gain=0.01  offset=-10
  VHAL_MELanePosRt2_m : Outport
  wires:
  convert_in/1 -> VHAL_MELanePosRt2_m/1
  UnitConverter/1 -> convert_in/1
  ME_Lane_PosRt2/1 -> UnitConverter/1

== system halin/HAL_IN/CAN6/SRR1/SRRBSDWarnL ==
  SRR_BSD_WarnL : Inport
  UnitConverter : DataTypeConversion  OutDataTypeStr=uint8
  VHAL_SRRBSDWarnL_enum : Outport
  wires:
  UnitConverter/1 -> VHAL_SRRBSDWarnL_enum/1
  SRR_BSD_WarnL/1 -> UnitConverter/1

== system halin/HAL_IN/CAN6/SRR1/SRRBSDWarnR ==
  SRR_BSD_WarnR : Inport
  UnitConverter : DataTypeConversion  OutDataTypeStr=uint8
  VHAL_SRRBSDWarnR_enum : Outport
  wires:
  UnitConverter/1 -> VHAL_SRRBSDWarnR_enum/1
  SRR_BSD_WarnR/1 -> UnitConverter/1

== system halin/HAL_IN/CAN6/SRR1/SRRODAWarnL ==
  SRR_ODA_WarnL : Inport
  UnitConverter : DataTypeConversion  OutDataTypeStr=uint8
  VHAL_SRRODAWarnL_enum : Outport
  wires:
  UnitConverter/1 -> VHAL_SRRODAWarnL_enum/1
  SRR_ODA_WarnL/1 -> UnitConverter/1

== system halin/HAL_IN/CAN6/SRR1/SRRODAWarnR ==
  SRR_ODA_WarnR : Inport
  UnitConverter : DataTypeConversion  OutDataTypeStr=uint8
  VHAL_SRRODAWarnR_enum : Outport
  wires:
  UnitConverter/1 -> VHAL_SRRODAWarnR_enum/1
  SRR_ODA_WarnR/1 -> UnitConverter/1
